simulink model "traffic_light_simple"  (R2025a)
settings: Solver=FixedStepAuto  StartTime=0.0  StopTime=20  FixedStep=0.5  RelTol=1e-3
settings Model: Creator=Issam  LastModifiedBy=Issam

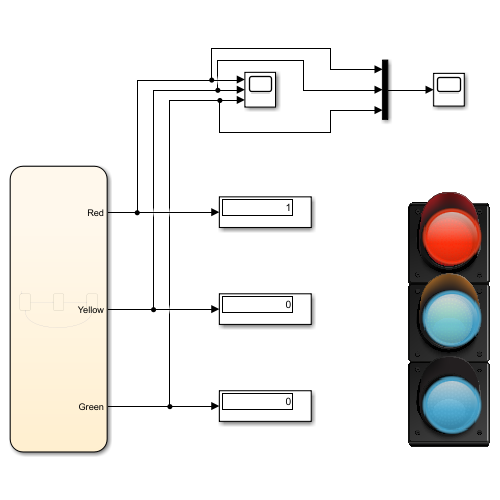
[thumbnail: Simulink's stored preview of the top-level diagram]
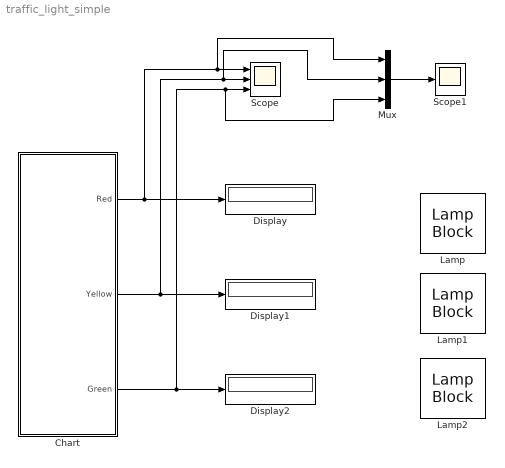
== system traffic_light_simple ==
  Chart : Stateflow chart  TreatAsAtomicUnit=on
  Display : Display
  Display1 : Display
  Display2 : Display
  Lamp : LampBlock  LabelPosition=Hide  DefaultColor=[77.0, 190.0, 238.0]
  Lamp1 : LampBlock  LabelPosition=Hide  DefaultColor=[77.0, 190.0, 238.0]
  Lamp2 : LampBlock  LabelPosition=Hide  DefaultColor=[77.0, 190.0, 238.0]
  Mux : Mux  Inputs=3
  Scope : Scope  NumInputPorts=3
      settings: ActiveDisplayString=3  ActiveDisplayYMinimum=-1  ActiveDisplayYMaximum=1
  Scope1 : Scope
      settings: ActiveDisplayYMinimum=-0.12499999999999997  ActiveDisplayYMaximum=1.125
  wires:
  Chart/1(Red) -> Mux/1, Scope/1, Display/1
  Chart/2(Yellow) -> Mux/2, Scope/2, Display1/1
  Chart/3(Green) -> Mux/3, Scope/3, Display2/1
  Mux/1 -> Scope1/1

== stateflow chart traffic_light_simple/Chart ==
  settings: sampleTime=1
  state Stop
    en:
    Red = 1;
    Yellow = 0;
    Green = 0;
  state Go
    en:
    Red = 0;
    Yellow = 0;
    Green = 1;
  state ReadyToStop
    en:
    Red = 0;
    Yellow = 1;
    Green = 0;
  (default) -> Stop
  Stop -> Go : after(3,sec)
  Go -> ReadyToStop : after(5,sec)
  ReadyToStop -> Stop : after(2,sec)
  data: Red output; Yellow output; Green output
